simulink library "motor_control_lib"  (R2023b)
settings: Solver=VariableStepAuto  StartTime=0.0  StopTime=10.0  RelTol=1e-3
values from neighbouring files (symbols this model uses):
  current_pi_simcfg = 5.0E-5    [motor_control_interface.sldd]
  DeadtimeCompCurrentInvRange_1perA = 12.5    [motor_control_interface.sldd]
  DeadtimeCompCurrentZero_A = 0.019999999552965164    [motor_control_interface.sldd]
  DeadtimeCompDuty = 0.0099999997764825821    [motor_control_interface.sldd]
  DeadtimeCompEnable = 1.0    [motor_control_interface.sldd]
  DeadtimeCompPolarity = -1.0    [motor_control_interface.sldd]
  inverter = 68.0    [motor_control_interface.sldd]
  Kaw_id = 400.0    [motor_control_interface.sldd]
  Kaw_iq = 400.0    [motor_control_interface.sldd]
  Kaw_speed = 40.0    [motor_control_interface.sldd]
  Ki_id = 1072.4140625    [motor_control_interface.sldd]
  Ki_iq = 1072.4140625    [motor_control_interface.sldd]
  Ki_speed = 79.284461975097656    [motor_control_interface.sldd]
  Kp_id = 1.3320353031158447    [motor_control_interface.sldd]
  Kp_iq = 1.3320353031158447    [motor_control_interface.sldd]
  Kp_speed = 0.63092565536499023    [motor_control_interface.sldd]
  openloop = 0.0    [motor_control_interface.sldd]
  simcfg = 0.06    [motor_control_interface.sldd]
  speed_pi_simcfg = 0.0001    [motor_control_interface.sldd]
  VLimitRatio = 0.57700002193450928    [motor_control_interface.sldd]
settings Model: Creator=user  LastModifiedBy=user

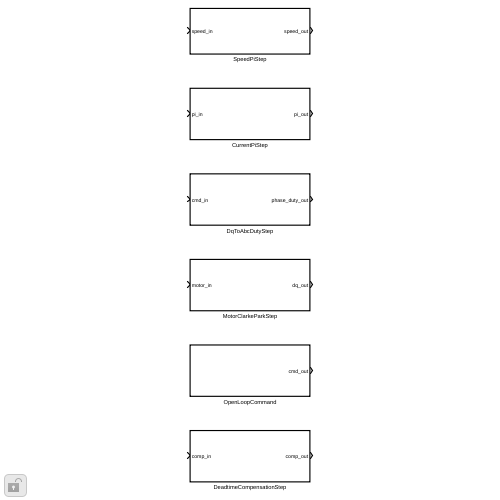
[thumbnail: Simulink's stored preview of the top-level diagram]
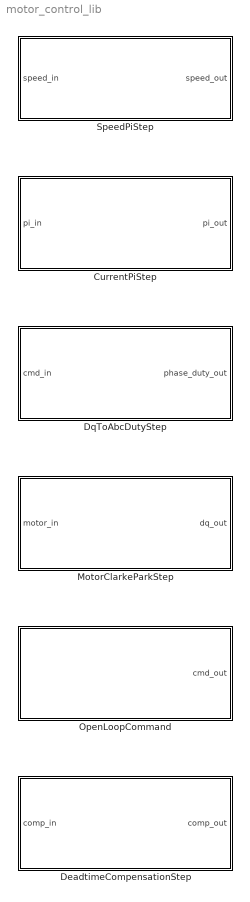
== system motor_control_lib ==
  CurrentPiStep : Subsystem  TreatAsAtomicUnit=on  RTWFcnName=CurrentPiStep  RTWFileName=CurrentPiStep
      settings: RTWFcnNameOpts=User specified  RTWFileNameOpts=User specified
  DeadtimeCompensationStep : Subsystem  TreatAsAtomicUnit=on  RTWFcnName=DeadtimeCompensationStep  RTWFileName=DeadtimeCompensationStep
      settings: RTWFcnNameOpts=User specified  RTWFileNameOpts=User specified
  DqToAbcDutyStep : Subsystem  TreatAsAtomicUnit=on  RTWFcnName=DqToAbcDutyStep  RTWFileName=DqToAbcDutyStep
      settings: RTWFcnNameOpts=User specified  RTWFileNameOpts=User specified
  MotorClarkeParkStep : Subsystem  TreatAsAtomicUnit=on  RTWFcnName=MotorClarkeParkStep  RTWFileName=MotorClarkeParkStep
      settings: RTWFcnNameOpts=User specified  RTWFileNameOpts=User specified
  OpenLoopCommand : Subsystem  TreatAsAtomicUnit=on  RTWFcnName=OpenLoopCommandStep  RTWFileName=OpenLoopCommandStep
      settings: RTWFcnNameOpts=User specified  RTWFileNameOpts=User specified
  SpeedPiStep : Subsystem  TreatAsAtomicUnit=on  RTWFcnName=SpeedPiStep  RTWFileName=SpeedPiStep
      settings: RTWFcnNameOpts=User specified  RTWFileNameOpts=User specified

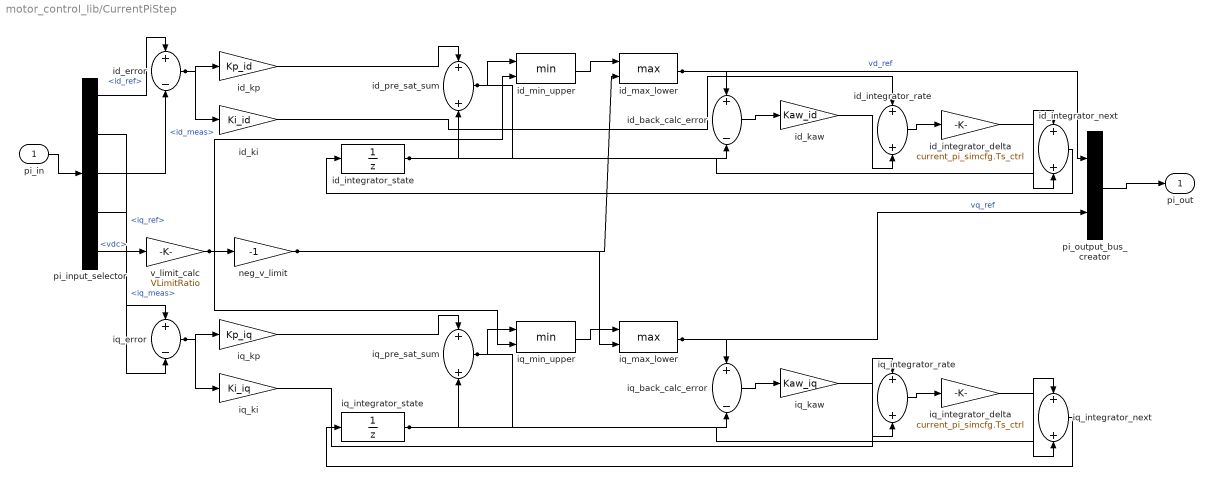
== system motor_control_lib/CurrentPiStep ==
  pi_in : Inport  OutDataTypeStr=Bus: current_pi_input_t  BusOutputAsStruct=on
  id_back_calc_error : Sum  Inputs=+-  OutDataTypeStr=T_CurrentPiVoltage  AccumDataTypeStr=T_CurrentPiVoltage
  id_error : Sum  Inputs=+-  OutDataTypeStr=T_CurrentPiCurrent  AccumDataTypeStr=T_CurrentPiCurrent
  id_integrator_delta : Gain  Gain=current_pi_simcfg.Ts_ctrl  ParamDataTypeStr=T_CurrentPiFloat  OutDataTypeStr=T_CurrentPiVoltage
  id_integrator_next : Sum  OutDataTypeStr=T_CurrentPiVoltage  AccumDataTypeStr=T_CurrentPiVoltage
  id_integrator_rate : Sum  OutDataTypeStr=T_CurrentPiVoltage  AccumDataTypeStr=T_CurrentPiVoltage
  id_integrator_state : UnitDelay  SampleTime=current_pi_simcfg.Ts_ctrl  HasFrameUpgradeWarning=on
  id_kaw : Gain  Gain=Kaw_id  ParamDataTypeStr=T_CurrentPiGain  OutDataTypeStr=T_CurrentPiVoltage
  id_ki : Gain  Gain=Ki_id  ParamDataTypeStr=T_CurrentPiGain  OutDataTypeStr=T_CurrentPiVoltage
  id_kp : Gain  Gain=Kp_id  ParamDataTypeStr=T_CurrentPiGain  OutDataTypeStr=T_CurrentPiVoltage
  id_max_lower : MinMax  Function=max  Inputs=2
  id_min_upper : MinMax  Inputs=2
  id_pre_sat_sum : Sum  OutDataTypeStr=T_CurrentPiVoltage  AccumDataTypeStr=T_CurrentPiVoltage
  iq_back_calc_error : Sum  Inputs=+-  OutDataTypeStr=T_CurrentPiVoltage  AccumDataTypeStr=T_CurrentPiVoltage
  iq_error : Sum  Inputs=+-  OutDataTypeStr=T_CurrentPiCurrent  AccumDataTypeStr=T_CurrentPiCurrent
  iq_integrator_delta : Gain  Gain=current_pi_simcfg.Ts_ctrl  ParamDataTypeStr=T_CurrentPiFloat  OutDataTypeStr=T_CurrentPiVoltage
  iq_integrator_next : Sum  OutDataTypeStr=T_CurrentPiVoltage  AccumDataTypeStr=T_CurrentPiVoltage
  iq_integrator_rate : Sum  OutDataTypeStr=T_CurrentPiVoltage  AccumDataTypeStr=T_CurrentPiVoltage
  iq_integrator_state : UnitDelay  SampleTime=current_pi_simcfg.Ts_ctrl  HasFrameUpgradeWarning=on
  iq_kaw : Gain  Gain=Kaw_iq  ParamDataTypeStr=T_CurrentPiGain  OutDataTypeStr=T_CurrentPiVoltage
  iq_ki : Gain  Gain=Ki_iq  ParamDataTypeStr=T_CurrentPiGain  OutDataTypeStr=T_CurrentPiVoltage
  iq_kp : Gain  Gain=Kp_iq  ParamDataTypeStr=T_CurrentPiGain  OutDataTypeStr=T_CurrentPiVoltage
  iq_max_lower : MinMax  Function=max  Inputs=2
  iq_min_upper : MinMax  Inputs=2
  iq_pre_sat_sum : Sum  OutDataTypeStr=T_CurrentPiVoltage  AccumDataTypeStr=T_CurrentPiVoltage
  neg_v_limit : Gain  Gain=-1  ParamDataTypeStr=T_CurrentPiFloat  OutDataTypeStr=T_CurrentPiVoltage
  pi_input_selector : BusSelector  OutputSignals=id_ref,iq_ref,id_meas,iq_meas,vdc
  pi_output_bus_creator : BusCreator  Inputs=2  OutDataTypeStr=Bus: current_pi_output_t  NonVirtualBus=on
  v_limit_calc : Gain  Gain=VLimitRatio  ParamDataTypeStr=T_CurrentPiGain  OutDataTypeStr=T_CurrentPiVoltage
  pi_out : Outport  OutDataTypeStr=Bus: current_pi_output_t
  wires:
  pi_output_bus_creator/1 -> pi_out/1
  iq_integrator_next/1 -> iq_integrator_state/1
  iq_integrator_delta/1 -> iq_integrator_next/2
  iq_integrator_rate/1 -> iq_integrator_delta/1
  iq_kaw/1 -> iq_integrator_rate/2
  iq_ki/1 -> iq_integrator_rate/1
  iq_back_calc_error/1 -> iq_kaw/1
  iq_max_lower/1 -> pi_output_bus_creator/2, iq_back_calc_error/1  "vq_ref"
  iq_min_upper/1 -> iq_max_lower/1
  iq_pre_sat_sum/1 -> iq_back_calc_error/2, iq_min_upper/1
  iq_integrator_state/1 -> iq_integrator_next/1, iq_pre_sat_sum/2
  iq_kp/1 -> iq_pre_sat_sum/1
  iq_error/1 -> iq_ki/1, iq_kp/1
  pi_input_selector/4 -> iq_error/2  "<iq_meas>"
  pi_input_selector/2 -> iq_error/1  "<iq_ref>"
  id_integrator_next/1 -> id_integrator_state/1
  id_integrator_delta/1 -> id_integrator_next/2
  id_integrator_rate/1 -> id_integrator_delta/1
  id_kaw/1 -> id_integrator_rate/2
  id_ki/1 -> id_integrator_rate/1
  id_back_calc_error/1 -> id_kaw/1
  id_max_lower/1 -> pi_output_bus_creator/1, id_back_calc_error/1  "vd_ref"
  neg_v_limit/1 -> iq_max_lower/2, id_max_lower/2
  id_min_upper/1 -> id_max_lower/1
  id_pre_sat_sum/1 -> id_back_calc_error/2, id_min_upper/1
  id_integrator_state/1 -> id_integrator_next/1, id_pre_sat_sum/2
  id_kp/1 -> id_pre_sat_sum/1
  id_error/1 -> id_ki/1, id_kp/1
  pi_input_selector/3 -> id_error/2  "<id_meas>"
  pi_input_selector/1 -> id_error/1  "<id_ref>"
  v_limit_calc/1 -> iq_min_upper/2, id_min_upper/2, neg_v_limit/1
  pi_input_selector/5 -> v_limit_calc/1  "<vdc>"
  pi_in/1 -> pi_input_selector/1

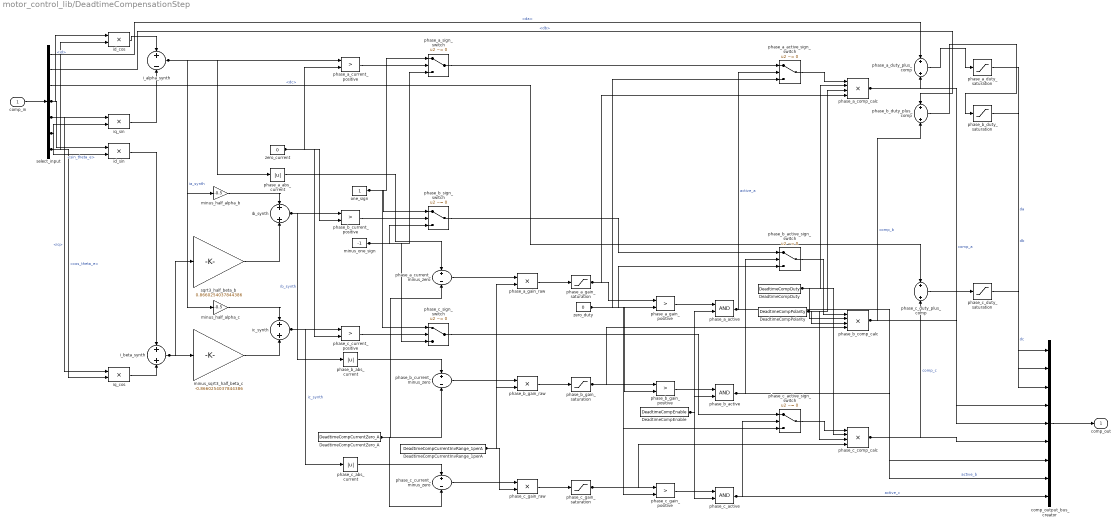
== system motor_control_lib/DeadtimeCompensationStep ==
  comp_in : Inport  OutDataTypeStr=Bus: pwm_deadtime_comp_input_t  PortDimensions=1  BusOutputAsStruct=on
  DeadtimeCompCurrentInvRange_1perA : Constant  Value=DeadtimeCompCurrentInvRange_1perA  OutDataTypeStr=T_DeadtimeCompDuty  SampleTime=-1
  DeadtimeCompCurrentZero_A : Constant  Value=DeadtimeCompCurrentZero_A  OutDataTypeStr=T_DeadtimeCompCurrent  SampleTime=-1
  DeadtimeCompDuty : Constant  Value=DeadtimeCompDuty  OutDataTypeStr=T_DeadtimeCompDuty  SampleTime=-1
  DeadtimeCompEnable : Constant  Value=DeadtimeCompEnable  OutDataTypeStr=T_DeadtimeCompBool  SampleTime=-1
  DeadtimeCompPolarity : Constant  Value=DeadtimeCompPolarity  OutDataTypeStr=T_DeadtimeCompDuty  SampleTime=-1
  comp_output_bus_creator : BusCreator  Inputs=9  OutDataTypeStr=Bus: pwm_deadtime_comp_output_t  NonVirtualBus=on
  i_alpha_synth : Sum  Inputs=+-  OutDataTypeStr=T_DeadtimeCompCurrent
  i_beta_synth : Sum  OutDataTypeStr=T_DeadtimeCompCurrent
  ib_synth : Sum  OutDataTypeStr=T_DeadtimeCompCurrent
  ic_synth : Sum  OutDataTypeStr=T_DeadtimeCompCurrent
  id_cos : Product  Inputs=**  OutDataTypeStr=T_DeadtimeCompCurrent
  id_sin : Product  Inputs=**  OutDataTypeStr=T_DeadtimeCompCurrent
  iq_cos : Product  Inputs=**  OutDataTypeStr=T_DeadtimeCompCurrent
  iq_sin : Product  Inputs=**  OutDataTypeStr=T_DeadtimeCompCurrent
  minus_half_alpha_b : Gain  Gain=-0.5  OutDataTypeStr=T_DeadtimeCompCurrent
  minus_half_alpha_c : Gain  Gain=-0.5  OutDataTypeStr=T_DeadtimeCompCurrent
  minus_one_sign : Constant  Value=-1  OutDataTypeStr=T_DeadtimeCompDuty  SampleTime=-1
  minus_sqrt3_half_beta_c : Gain  Gain=-0.8660254037844386  OutDataTypeStr=T_DeadtimeCompCurrent
  one_sign : Constant  OutDataTypeStr=T_DeadtimeCompDuty  SampleTime=-1
  phase_a_abs_current : Abs  SaturateOnIntegerOverflow=off
  phase_a_active : Logic  AllPortsSameDT=off  OutDataTypeStr=T_DeadtimeCompBool
  phase_a_active_sign_switch : Switch  Criteria=u2 ~= 0  OutDataTypeStr=T_DeadtimeCompDuty  SaturateOnIntegerOverflow=off  InputSameDT=off
  phase_a_comp_calc : Product  Inputs=****  OutDataTypeStr=T_DeadtimeCompDuty
  phase_a_current_minus_zero : Sum  Inputs=+-  OutDataTypeStr=T_DeadtimeCompCurrent
  phase_a_current_positive : RelationalOperator  Operator=>  OutDataTypeStr=boolean  RndMeth=Simplest  InputSameDT=off
  phase_a_duty_plus_comp : Sum  OutDataTypeStr=T_DeadtimeCompDuty
  phase_a_duty_saturation : Saturate  UpperLimit=1  LowerLimit=0  OutDataTypeStr=T_DeadtimeCompDuty
  phase_a_gain_positive : RelationalOperator  Operator=>  OutDataTypeStr=boolean  RndMeth=Simplest  InputSameDT=off
  phase_a_gain_raw : Product  Inputs=**  OutDataTypeStr=T_DeadtimeCompDuty
  phase_a_gain_saturation : Saturate  UpperLimit=1  LowerLimit=0  OutDataTypeStr=T_DeadtimeCompDuty
  phase_a_sign_switch : Switch  Criteria=u2 ~= 0  OutDataTypeStr=T_DeadtimeCompDuty  SaturateOnIntegerOverflow=off  InputSameDT=off
  phase_b_abs_current : Abs  SaturateOnIntegerOverflow=off
  phase_b_active : Logic  AllPortsSameDT=off  OutDataTypeStr=T_DeadtimeCompBool
  phase_b_active_sign_switch : Switch  Criteria=u2 ~= 0  OutDataTypeStr=T_DeadtimeCompDuty  SaturateOnIntegerOverflow=off  InputSameDT=off
  phase_b_comp_calc : Product  Inputs=****  OutDataTypeStr=T_DeadtimeCompDuty
  phase_b_current_minus_zero : Sum  Inputs=+-  OutDataTypeStr=T_DeadtimeCompCurrent
  phase_b_current_positive : RelationalOperator  Operator=>  OutDataTypeStr=boolean  RndMeth=Simplest  InputSameDT=off
  phase_b_duty_plus_comp : Sum  OutDataTypeStr=T_DeadtimeCompDuty
  phase_b_duty_saturation : Saturate  UpperLimit=1  LowerLimit=0  OutDataTypeStr=T_DeadtimeCompDuty
  phase_b_gain_positive : RelationalOperator  Operator=>  OutDataTypeStr=boolean  RndMeth=Simplest  InputSameDT=off
  phase_b_gain_raw : Product  Inputs=**  OutDataTypeStr=T_DeadtimeCompDuty
  phase_b_gain_saturation : Saturate  UpperLimit=1  LowerLimit=0  OutDataTypeStr=T_DeadtimeCompDuty
  phase_b_sign_switch : Switch  Criteria=u2 ~= 0  OutDataTypeStr=T_DeadtimeCompDuty  SaturateOnIntegerOverflow=off  InputSameDT=off
  phase_c_abs_current : Abs  SaturateOnIntegerOverflow=off
  phase_c_active : Logic  AllPortsSameDT=off  OutDataTypeStr=T_DeadtimeCompBool
  phase_c_active_sign_switch : Switch  Criteria=u2 ~= 0  OutDataTypeStr=T_DeadtimeCompDuty  SaturateOnIntegerOverflow=off  InputSameDT=off
  phase_c_comp_calc : Product  Inputs=****  OutDataTypeStr=T_DeadtimeCompDuty
  phase_c_current_minus_zero : Sum  Inputs=+-  OutDataTypeStr=T_DeadtimeCompCurrent
  phase_c_current_positive : RelationalOperator  Operator=>  OutDataTypeStr=boolean  RndMeth=Simplest  InputSameDT=off
  phase_c_duty_plus_comp : Sum  OutDataTypeStr=T_DeadtimeCompDuty
  phase_c_duty_saturation : Saturate  UpperLimit=1  LowerLimit=0  OutDataTypeStr=T_DeadtimeCompDuty
  phase_c_gain_positive : RelationalOperator  Operator=>  OutDataTypeStr=boolean  RndMeth=Simplest  InputSameDT=off
  phase_c_gain_raw : Product  Inputs=**  OutDataTypeStr=T_DeadtimeCompDuty
  phase_c_gain_saturation : Saturate  UpperLimit=1  LowerLimit=0  OutDataTypeStr=T_DeadtimeCompDuty
  phase_c_sign_switch : Switch  Criteria=u2 ~= 0  OutDataTypeStr=T_DeadtimeCompDuty  SaturateOnIntegerOverflow=off  InputSameDT=off
  select_input : BusSelector  OutputSignals=da,db,dc,id,iq,sin_theta_e,cos_theta_e
  sqrt3_half_beta_b : Gain  Gain=0.8660254037844386  OutDataTypeStr=T_DeadtimeCompCurrent
  zero_current : Constant  Value=0  OutDataTypeStr=T_DeadtimeCompCurrent  SampleTime=-1
  zero_duty : Constant  Value=0  OutDataTypeStr=T_DeadtimeCompDuty  SampleTime=-1
  comp_out : Outport  OutDataTypeStr=Bus: pwm_deadtime_comp_output_t  PortDimensions=1
  wires:
  phase_b_comp_calc/1 -> comp_output_bus_creator/5, phase_b_duty_plus_comp/2  "comp_b"
  phase_b_active_sign_switch/1 -> phase_b_comp_calc/1
  phase_a_gain_positive/1 -> phase_a_active/1
  phase_b_gain_saturation/1 -> phase_b_comp_calc/4, phase_b_gain_positive/1
  phase_c_gain_positive/1 -> phase_c_active/1
  minus_sqrt3_half_beta_c/1 -> ic_synth/2
  zero_duty/1 -> phase_b_active_sign_switch/3, phase_c_gain_positive/2, phase_c_active_sign_switch/3, phase_a_active_sign_switch/3, phase_a_gain_positive/2, phase_b_gain_positive/2
  phase_c_gain_raw/1 -> phase_c_gain_saturation/1
  phase_a_gain_saturation/1 -> phase_a_comp_calc/4, phase_a_gain_positive/1
  phase_b_gain_raw/1 -> phase_b_gain_saturation/1
  phase_a_gain_raw/1 -> phase_a_gain_saturation/1
  select_input/1 -> phase_a_duty_plus_comp/1  "<da>"
  phase_c_current_minus_zero/1 -> phase_c_gain_raw/1
  phase_c_duty_plus_comp/1 -> phase_c_duty_saturation/1
  DeadtimeCompCurrentInvRange_1perA/1 -> phase_a_gain_raw/2, phase_c_gain_raw/2, phase_b_gain_raw/2
  minus_half_alpha_b/1 -> ib_synth/1
  phase_a_active_sign_switch/1 -> phase_a_comp_calc/1
  phase_b_sign_switch/1 -> phase_b_active_sign_switch/1
  phase_c_comp_calc/1 -> comp_output_bus_creator/6, phase_c_duty_plus_comp/2  "comp_c"
  phase_a_sign_switch/1 -> phase_a_active_sign_switch/1
  phase_c_abs_current/1 -> phase_c_current_minus_zero/1
  phase_c_sign_switch/1 -> phase_c_active_sign_switch/1
  id_sin/1 -> i_beta_synth/1
  id_cos/1 -> i_alpha_synth/1
  select_input/7 -> id_cos/2, iq_cos/2  "<cos_theta_e>"
  zero_current/1 -> phase_a_current_positive/2, phase_c_current_positive/2, phase_b_current_positive/2
  phase_b_current_minus_zero/1 -> phase_b_gain_raw/1
  select_input/6 -> iq_sin/2, id_sin/2  "<sin_theta_e>"
  phase_c_active_sign_switch/1 -> phase_c_comp_calc/1
  comp_in/1 -> select_input/1
  DeadtimeCompPolarity/1 -> phase_c_comp_calc/3, phase_a_comp_calc/3, phase_b_comp_calc/3
  select_input/4 -> id_cos/1, id_sin/1  "<id>"
  i_alpha_synth/1 -> phase_a_current_positive/1, minus_half_alpha_b/1, phase_a_abs_current/1, minus_half_alpha_c/1  "ia_synth"
  phase_a_active/1 -> comp_output_bus_creator/7, phase_a_active_sign_switch/2  "active_a"
  phase_a_comp_calc/1 -> comp_output_bus_creator/4, phase_a_duty_plus_comp/2  "comp_a"
  phase_c_active/1 -> comp_output_bus_creator/9, phase_c_active_sign_switch/2  "active_c"
  phase_b_active/1 -> comp_output_bus_creator/8, phase_b_active_sign_switch/2  "active_b"
  iq_cos/1 -> i_beta_synth/2
  DeadtimeCompEnable/1 -> phase_a_active/2, phase_c_active/2, phase_b_active/2
  phase_b_abs_current/1 -> phase_b_current_minus_zero/1
  select_input/3 -> phase_c_duty_plus_comp/1  "<dc>"
  DeadtimeCompDuty/1 -> phase_a_comp_calc/2, phase_c_comp_calc/2, phase_b_comp_calc/2
  iq_sin/1 -> i_alpha_synth/2
  i_beta_synth/1 -> sqrt3_half_beta_b/1, minus_sqrt3_half_beta_c/1
  phase_c_gain_saturation/1 -> phase_c_comp_calc/4, phase_c_gain_positive/1
  phase_a_abs_current/1 -> phase_a_current_minus_zero/1
  ic_synth/1 -> phase_c_abs_current/1, phase_c_current_positive/1  "ic_synth"
  select_input/5 -> iq_sin/1, iq_cos/1  "<iq>"
  phase_c_duty_saturation/1 -> comp_output_bus_creator/3  "dc"
  minus_one_sign/1 -> phase_a_sign_switch/3, phase_c_sign_switch/3, phase_b_sign_switch/3
  phase_b_gain_positive/1 -> phase_b_active/1
  phase_a_current_minus_zero/1 -> phase_a_gain_raw/1
  one_sign/1 -> phase_c_sign_switch/1, phase_a_sign_switch/1, phase_b_sign_switch/1
  sqrt3_half_beta_b/1 -> ib_synth/2
  minus_half_alpha_c/1 -> ic_synth/1
  select_input/2 -> phase_b_duty_plus_comp/1  "<db>"
  phase_b_current_positive/1 -> phase_b_sign_switch/2
  phase_c_current_positive/1 -> phase_c_sign_switch/2
  phase_a_current_positive/1 -> phase_a_sign_switch/2
  ib_synth/1 -> phase_b_abs_current/1, phase_b_current_positive/1  "ib_synth"
  DeadtimeCompCurrentZero_A/1 -> phase_c_current_minus_zero/2, phase_b_current_minus_zero/2, phase_a_current_minus_zero/2
  phase_a_duty_plus_comp/1 -> phase_a_duty_saturation/1
  phase_b_duty_plus_comp/1 -> phase_b_duty_saturation/1
  phase_a_duty_saturation/1 -> comp_output_bus_creator/1  "da"
  phase_b_duty_saturation/1 -> comp_output_bus_creator/2  "db"
  comp_output_bus_creator/1 -> comp_out/1

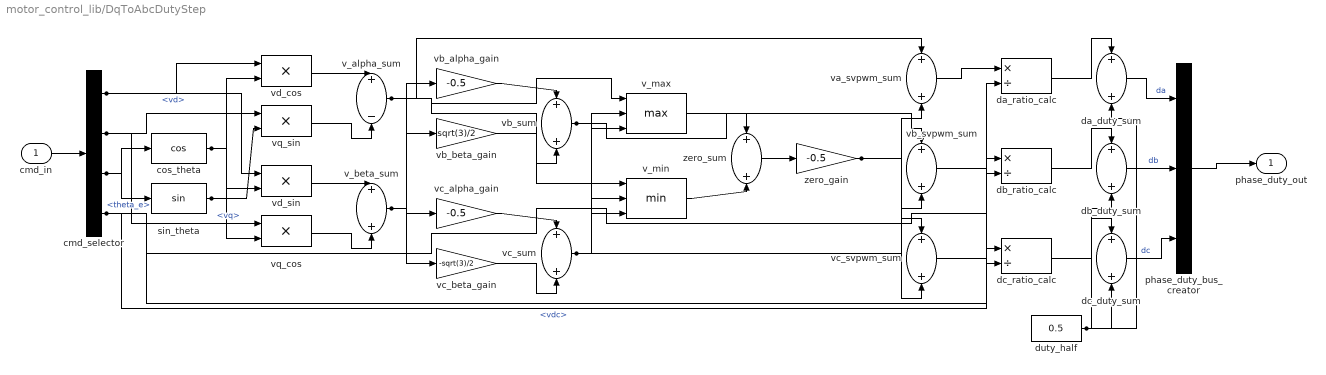
== system motor_control_lib/DqToAbcDutyStep ==
  cmd_in : Inport  OutDataTypeStr=Bus: open_loop_cmd_t  BusOutputAsStruct=on
  cmd_selector : BusSelector  OutputSignals=vd,vq,theta_e,vdc
  cos_theta : Trigonometry  Operator=cos
  da_duty_sum : Sum  OutDataTypeStr=T_DutyRatio  AccumDataTypeStr=T_DutyRatio
  da_ratio_calc : Product  Inputs=*/  OutDataTypeStr=T_DutyRatio
  db_duty_sum : Sum  OutDataTypeStr=T_DutyRatio  AccumDataTypeStr=T_DutyRatio
  db_ratio_calc : Product  Inputs=*/  OutDataTypeStr=T_DutyRatio
  dc_duty_sum : Sum  OutDataTypeStr=T_DutyRatio  AccumDataTypeStr=T_DutyRatio
  dc_ratio_calc : Product  Inputs=*/  OutDataTypeStr=T_DutyRatio
  duty_half : Constant  Value=0.5  OutDataTypeStr=T_DutyRatio  SampleTime=simcfg.Ts_ctrl
  phase_duty_bus_creator : BusCreator  Inputs=3  OutDataTypeStr=Bus: phase_duty_t  NonVirtualBus=on
  sin_theta : Trigonometry
  v_alpha_sum : Sum  Inputs=+-  OutDataTypeStr=T_MotorVoltage  AccumDataTypeStr=T_MotorVoltage
  v_beta_sum : Sum  OutDataTypeStr=T_MotorVoltage  AccumDataTypeStr=T_MotorVoltage
  v_max : MinMax  Function=max  Inputs=3
  v_min : MinMax  Inputs=3
  va_svpwm_sum : Sum  OutDataTypeStr=T_MotorVoltage  AccumDataTypeStr=T_MotorVoltage
  vb_alpha_gain : Gain  Gain=-0.5  ParamDataTypeStr=T_MotorFloat  OutDataTypeStr=T_MotorVoltage
  vb_beta_gain : Gain  Gain=sqrt(3)/2  ParamDataTypeStr=T_MotorFloat  OutDataTypeStr=T_MotorVoltage
  vb_sum : Sum  OutDataTypeStr=T_MotorVoltage  AccumDataTypeStr=T_MotorVoltage
  vb_svpwm_sum : Sum  OutDataTypeStr=T_MotorVoltage  AccumDataTypeStr=T_MotorVoltage
  vc_alpha_gain : Gain  Gain=-0.5  ParamDataTypeStr=T_MotorFloat  OutDataTypeStr=T_MotorVoltage
  vc_beta_gain : Gain  Gain=-sqrt(3)/2  ParamDataTypeStr=T_MotorFloat  OutDataTypeStr=T_MotorVoltage
  vc_sum : Sum  OutDataTypeStr=T_MotorVoltage  AccumDataTypeStr=T_MotorVoltage
  vc_svpwm_sum : Sum  OutDataTypeStr=T_MotorVoltage  AccumDataTypeStr=T_MotorVoltage
  vd_cos : Product  Inputs=**  OutDataTypeStr=T_MotorVoltage
  vd_sin : Product  Inputs=**  OutDataTypeStr=T_MotorVoltage
  vq_cos : Product  Inputs=**  OutDataTypeStr=T_MotorVoltage
  vq_sin : Product  Inputs=**  OutDataTypeStr=T_MotorVoltage
  zero_gain : Gain  Gain=-0.5  ParamDataTypeStr=T_MotorFloat  OutDataTypeStr=T_MotorVoltage
  zero_sum : Sum  OutDataTypeStr=T_MotorVoltage  AccumDataTypeStr=T_MotorVoltage
  phase_duty_out : Outport  OutDataTypeStr=Bus: phase_duty_t
  wires:
  phase_duty_bus_creator/1 -> phase_duty_out/1
  dc_duty_sum/1 -> phase_duty_bus_creator/3  "dc"
  db_duty_sum/1 -> phase_duty_bus_creator/2  "db"
  da_duty_sum/1 -> phase_duty_bus_creator/1  "da"
  duty_half/1 -> dc_duty_sum/2, db_duty_sum/2, da_duty_sum/2
  dc_ratio_calc/1 -> dc_duty_sum/1
  db_ratio_calc/1 -> db_duty_sum/1
  da_ratio_calc/1 -> da_duty_sum/1
  vc_svpwm_sum/1 -> dc_ratio_calc/1
  vb_svpwm_sum/1 -> db_ratio_calc/1
  cmd_selector/4 -> dc_ratio_calc/2, db_ratio_calc/2, da_ratio_calc/2  "<vdc>"
  va_svpwm_sum/1 -> da_ratio_calc/1
  zero_gain/1 -> vc_svpwm_sum/2, vb_svpwm_sum/2, va_svpwm_sum/2
  zero_sum/1 -> zero_gain/1
  v_min/1 -> zero_sum/2
  v_max/1 -> zero_sum/1
  vc_sum/1 -> vc_svpwm_sum/1, v_min/3, v_max/3
  vb_sum/1 -> vb_svpwm_sum/1, v_min/2, v_max/2
  vc_beta_gain/1 -> vc_sum/2
  vc_alpha_gain/1 -> vc_sum/1
  vb_beta_gain/1 -> vb_sum/2
  vb_alpha_gain/1 -> vb_sum/1
  v_beta_sum/1 -> vc_beta_gain/1, vb_beta_gain/1
  v_alpha_sum/1 -> va_svpwm_sum/1, v_min/1, v_max/1, vc_alpha_gain/1, vb_alpha_gain/1
  vq_cos/1 -> v_beta_sum/2
  vd_sin/1 -> v_beta_sum/1
  vq_sin/1 -> v_alpha_sum/2
  vd_cos/1 -> v_alpha_sum/1
  sin_theta/1 -> vd_sin/2, vq_sin/2
  cmd_selector/2 -> vq_cos/1, vq_sin/1  "<vq>"
  cos_theta/1 -> vq_cos/2, vd_cos/2
  cmd_selector/1 -> vd_sin/1, vd_cos/1  "<vd>"
  cmd_selector/3 -> sin_theta/1, cos_theta/1  "<theta_e>"
  cmd_in/1 -> cmd_selector/1

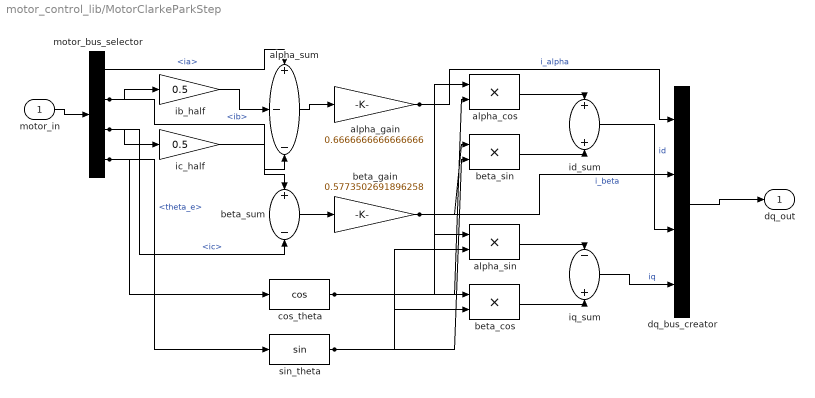
== system motor_control_lib/MotorClarkeParkStep ==
  motor_in : Inport  OutDataTypeStr=Bus: motor_t  BusOutputAsStruct=on
  alpha_cos : Product  Inputs=**  OutDataTypeStr=T_MotorCurrent  SaturateOnIntegerOverflow=on
  alpha_gain : Gain  Gain=0.6666666666666666  ParamDataTypeStr=T_MotorCurrent  OutDataTypeStr=T_MotorCurrent  SaturateOnIntegerOverflow=on
  alpha_sin : Product  Inputs=**  OutDataTypeStr=T_MotorCurrent  SaturateOnIntegerOverflow=on
  alpha_sum : Sum  Inputs=+--  OutDataTypeStr=T_MotorCurrent  AccumDataTypeStr=T_MotorCurrent  SaturateOnIntegerOverflow=on
  beta_cos : Product  Inputs=**  OutDataTypeStr=T_MotorCurrent  SaturateOnIntegerOverflow=on
  beta_gain : Gain  Gain=0.5773502691896258  ParamDataTypeStr=T_MotorCurrent  OutDataTypeStr=T_MotorCurrent  SaturateOnIntegerOverflow=on
  beta_sin : Product  Inputs=**  OutDataTypeStr=T_MotorCurrent  SaturateOnIntegerOverflow=on
  beta_sum : Sum  Inputs=+-  OutDataTypeStr=T_MotorCurrent  AccumDataTypeStr=T_MotorCurrent  SaturateOnIntegerOverflow=on
  cos_theta : Trigonometry  Operator=cos
  dq_bus_creator : BusCreator  Inputs=4  OutDataTypeStr=Bus: motor_dq_t  NonVirtualBus=on
  ib_half : Gain  Gain=0.5  ParamDataTypeStr=T_MotorCurrent  OutDataTypeStr=T_MotorCurrent  SaturateOnIntegerOverflow=on
  ic_half : Gain  Gain=0.5  ParamDataTypeStr=T_MotorCurrent  OutDataTypeStr=T_MotorCurrent  SaturateOnIntegerOverflow=on
  id_sum : Sum  OutDataTypeStr=T_MotorCurrent  AccumDataTypeStr=T_MotorCurrent  SaturateOnIntegerOverflow=on
  iq_sum : Sum  Inputs=-+  OutDataTypeStr=T_MotorCurrent  AccumDataTypeStr=T_MotorCurrent  SaturateOnIntegerOverflow=on
  motor_bus_selector : BusSelector  OutputSignals=ia,ib,ic,theta_e
  sin_theta : Trigonometry
  dq_out : Outport  OutDataTypeStr=Bus: motor_dq_t
  wires:
  dq_bus_creator/1 -> dq_out/1
  iq_sum/1 -> dq_bus_creator/4  "iq"
  id_sum/1 -> dq_bus_creator/3  "id"
  beta_cos/1 -> iq_sum/2
  alpha_sin/1 -> iq_sum/1
  beta_sin/1 -> id_sum/2
  alpha_cos/1 -> id_sum/1
  sin_theta/1 -> alpha_sin/2, beta_sin/2
  beta_gain/1 -> dq_bus_creator/2, beta_cos/1, beta_sin/1  "i_beta"
  cos_theta/1 -> beta_cos/2, alpha_cos/2
  alpha_gain/1 -> dq_bus_creator/1, alpha_sin/1, alpha_cos/1  "i_alpha"
  motor_bus_selector/4 -> sin_theta/1, cos_theta/1  "<theta_e>"
  beta_sum/1 -> beta_gain/1
  alpha_sum/1 -> alpha_gain/1
  ic_half/1 -> alpha_sum/3
  ib_half/1 -> alpha_sum/2
  motor_bus_selector/3 -> beta_sum/2, ic_half/1  "<ic>"
  motor_bus_selector/2 -> beta_sum/1, ib_half/1  "<ib>"
  motor_bus_selector/1 -> alpha_sum/1  "<ia>"
  motor_in/1 -> motor_bus_selector/1

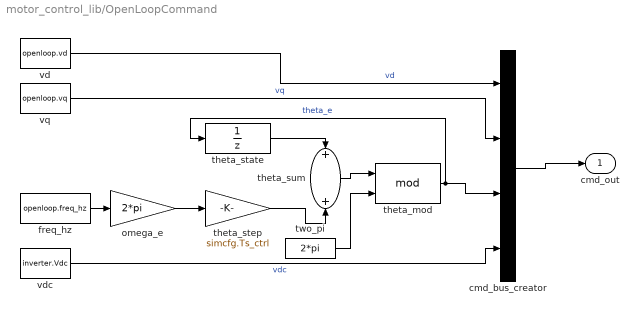
== system motor_control_lib/OpenLoopCommand ==
  cmd_bus_creator : BusCreator  Inputs=4  OutDataTypeStr=Bus: open_loop_cmd_t  NonVirtualBus=on
  freq_hz : Constant  Value=openloop.freq_hz  OutDataTypeStr=T_MotorFloat  SampleTime=simcfg.Ts_ctrl
  omega_e : Gain  Gain=2*pi  ParamDataTypeStr=T_MotorFloat  OutDataTypeStr=T_MotorFloat
  theta_mod : Math  Operator=mod  OutDataTypeStr=T_MotorAngle
  theta_state : UnitDelay  SampleTime=simcfg.Ts_ctrl  HasFrameUpgradeWarning=on
  theta_step : Gain  Gain=simcfg.Ts_ctrl  ParamDataTypeStr=T_MotorFloat  OutDataTypeStr=T_MotorAngle
  theta_sum : Sum  OutDataTypeStr=T_MotorAngle  AccumDataTypeStr=T_MotorAngle
  two_pi : Constant  Value=2*pi  OutDataTypeStr=T_MotorAngle  SampleTime=simcfg.Ts_ctrl
  vd : Constant  Value=openloop.vd  OutDataTypeStr=T_MotorVoltage  SampleTime=simcfg.Ts_ctrl
  vdc : Constant  Value=inverter.Vdc  OutDataTypeStr=T_MotorVoltage  SampleTime=simcfg.Ts_ctrl
  vq : Constant  Value=openloop.vq  OutDataTypeStr=T_MotorVoltage  SampleTime=simcfg.Ts_ctrl
  cmd_out : Outport  OutDataTypeStr=Bus: open_loop_cmd_t
  wires:
  cmd_bus_creator/1 -> cmd_out/1
  vdc/1 -> cmd_bus_creator/4  "vdc"
  vq/1 -> cmd_bus_creator/2  "vq"
  vd/1 -> cmd_bus_creator/1  "vd"
  theta_mod/1 -> cmd_bus_creator/3, theta_state/1  "theta_e"
  two_pi/1 -> theta_mod/2
  theta_sum/1 -> theta_mod/1
  theta_step/1 -> theta_sum/2
  theta_state/1 -> theta_sum/1
  omega_e/1 -> theta_step/1
  freq_hz/1 -> omega_e/1

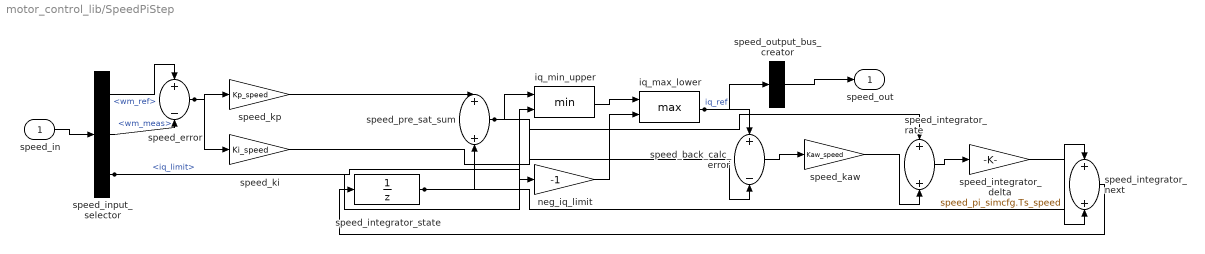
== system motor_control_lib/SpeedPiStep ==
  speed_in : Inport  OutDataTypeStr=Bus: speed_pi_input_t  BusOutputAsStruct=on
  iq_max_lower : MinMax  Function=max  Inputs=2
  iq_min_upper : MinMax  Inputs=2
  neg_iq_limit : Gain  Gain=-1  ParamDataTypeStr=T_SpeedPiFloat  OutDataTypeStr=T_SpeedPiCurrent
  speed_back_calc_error : Sum  Inputs=+-  OutDataTypeStr=T_SpeedPiCurrent  AccumDataTypeStr=T_SpeedPiCurrent
  speed_error : Sum  Inputs=+-  OutDataTypeStr=T_SpeedPiSpeed  AccumDataTypeStr=T_SpeedPiSpeed
  speed_input_selector : BusSelector  OutputSignals=wm_ref,wm_meas,iq_limit
  speed_integrator_delta : Gain  Gain=speed_pi_simcfg.Ts_speed  ParamDataTypeStr=T_SpeedPiFloat  OutDataTypeStr=T_SpeedPiCurrent
  speed_integrator_next : Sum  OutDataTypeStr=T_SpeedPiCurrent  AccumDataTypeStr=T_SpeedPiCurrent
  speed_integrator_rate : Sum  OutDataTypeStr=T_SpeedPiCurrent  AccumDataTypeStr=T_SpeedPiCurrent
  speed_integrator_state : UnitDelay  SampleTime=speed_pi_simcfg.Ts_speed  HasFrameUpgradeWarning=on
  speed_kaw : Gain  Gain=Kaw_speed  ParamDataTypeStr=T_SpeedPiGain  OutDataTypeStr=T_SpeedPiCurrent
  speed_ki : Gain  Gain=Ki_speed  ParamDataTypeStr=T_SpeedPiGain  OutDataTypeStr=T_SpeedPiCurrent
  speed_kp : Gain  Gain=Kp_speed  ParamDataTypeStr=T_SpeedPiGain  OutDataTypeStr=T_SpeedPiCurrent
  speed_output_bus_creator : BusCreator  Inputs=1  OutDataTypeStr=Bus: speed_pi_output_t  NonVirtualBus=on
  speed_pre_sat_sum : Sum  OutDataTypeStr=T_SpeedPiCurrent  AccumDataTypeStr=T_SpeedPiCurrent
  speed_out : Outport  OutDataTypeStr=Bus: speed_pi_output_t
  wires:
  speed_integrator_next/1 -> speed_integrator_state/1
  speed_integrator_delta/1 -> speed_integrator_next/2
  speed_integrator_rate/1 -> speed_integrator_delta/1
  speed_kaw/1 -> speed_integrator_rate/2
  speed_ki/1 -> speed_integrator_rate/1
  speed_back_calc_error/1 -> speed_kaw/1
  speed_output_bus_creator/1 -> speed_out/1
  iq_max_lower/1 -> speed_back_calc_error/1, speed_output_bus_creator/1  "iq_ref"
  neg_iq_limit/1 -> iq_max_lower/2
  iq_min_upper/1 -> iq_max_lower/1
  speed_input_selector/3 -> neg_iq_limit/1, iq_min_upper/2  "<iq_limit>"
  speed_pre_sat_sum/1 -> speed_back_calc_error/2, iq_min_upper/1
  speed_integrator_state/1 -> speed_integrator_next/1, speed_pre_sat_sum/2
  speed_kp/1 -> speed_pre_sat_sum/1
  speed_error/1 -> speed_ki/1, speed_kp/1
  speed_input_selector/2 -> speed_error/2  "<wm_meas>"
  speed_input_selector/1 -> speed_error/1  "<wm_ref>"
  speed_in/1 -> speed_input_selector/1
